simulink model "test_moteur"  (R2018a)
settings: Solver=FixedStepAuto  StartTime=0.0  StopTime=10.0  FixedStep=1e-5  RelTol=1e-3
values from neighbouring files (symbols this model uses):
  J = 0.0849    [datacn.mat]    (also in model.m = 0.0948)
  L = 0.00062    [datacn.mat]
  m = 2.1    [model.m]
undefined symbols (not defined in the file or in its folder): b, Cz, Kb, Kt, La, Ra, rho, S
settings Model: Creator=Maxence  LastModifiedBy=Maxence

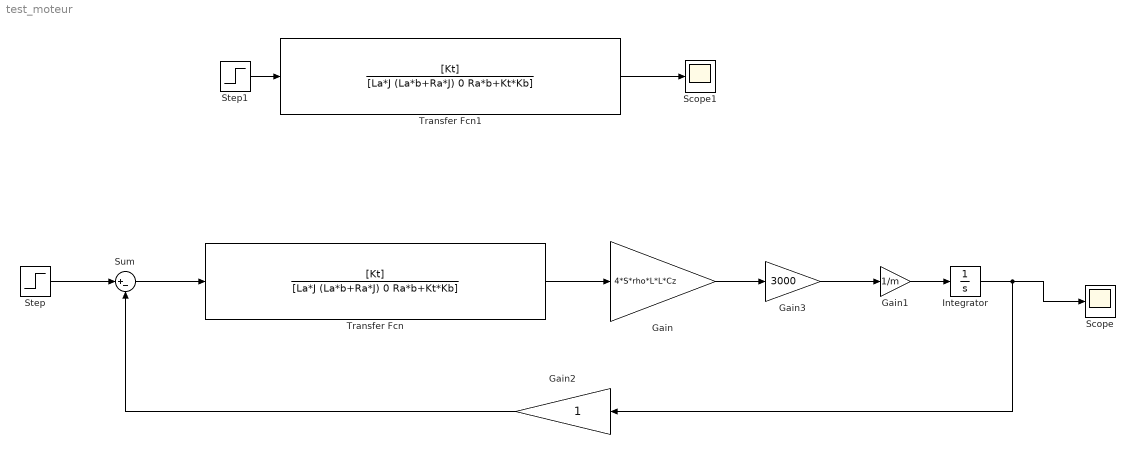
== system test_moteur ==
  Gain : Gain  Gain=4*S*rho*L*L*Cz
  Gain1 : Gain  Gain=1/m
  Gain2 : Gain
  Gain3 : Gain  Gain=3000
  Integrator : Integrator
  Scope : Scope
  Scope1 : Scope
  Step : Step  SampleTime=0
  Step1 : Step  SampleTime=0
  Sum : Sum  Inputs=|+-
  Transfer Fcn : TransferFcn  Numerator=[Kt]  Denominator=[La*J (La*b+Ra*J) 0 Ra*b+Kt*Kb]
  Transfer Fcn1 : TransferFcn  Numerator=[Kt]  Denominator=[La*J (La*b+Ra*J) 0 Ra*b+Kt*Kb]
  wires:
  Gain/1 -> Gain3/1
  Gain3/1 -> Gain1/1
  Sum/1 -> Transfer Fcn/1
  Gain2/1 -> Sum/2
  Gain1/1 -> Integrator/1
  Transfer Fcn/1 -> Gain/1
  Integrator/1 -> Scope/1, Gain2/1
  Step/1 -> Sum/1
  Step1/1 -> Transfer Fcn1/1
  Transfer Fcn1/1 -> Scope1/1
